simulink model "Traj_Track_twoDrones_CraneFast_ColAvo_2015b"  (R2015b)
settings: Solver=ode1  StartTime=0.0  StopTime=inf  FixedStep=T  RelTol=1e-3
StartFcn:
  | close all;
model workspace (MATLAB code in the model file):
  | T = .02; % simulation time step
values from neighbouring files (symbols this model uses):
  InitialPos_V1 = [-1 ; -1]    [CraneParam.m]
  LandFilter = ss(tf(0.3,[1 0.3]))    [CraneParam.m]
  pos_sat = 2.5    [CraneParam.m]
  radius_safe = 0.75    [CraneParam.m]
  repulsion_gain = 3.0    (= 3)    [CraneParam.m]
  repulsion_gradient = 0.2    [CraneParam.m]
  V1_gain = 0.25    [CraneParam.m]
undefined symbols (not defined in the file or in its folder): Angular, Linear, Point
libraries: robotlib x9, simulink x2, aerolibanimutils x1
settings Model: Creator=cichell2  LastModifiedBy=rmjones7
settings DataIOCC: LimitDataPoints=off  SaveFormat=Array  ReturnWorkspaceOutputs=on
settings OptimizationCC: OptimizeModelRefInitCode=on  LifeSpan=Inf  MaxStackSize=64
settings DebuggingCC: SolverPrmCheckMsg=warning
settings HardwareCC: ProdBitPerPointer=32  ProdLargestAtomicFloat=None  ProdIntDivRoundTo=Undefined  ProdEndianess=Unspecified  ProdWordSize=32  ProdHWDeviceType=Generic->Unspecified (assume 32-bit Generic)
settings RTWCC: SystemTargetFile=ert.tlc  TemplateMakefile=ert_default_tmf  Description=Embedded Coder  Toolchain=Catkin  TargetLang=C++
settings CodeAppCC: IgnoreCustomStorageClasses=off
settings ERTTargetCC: SupportContinuousTime=on
settings ConfigComp: CovModelRefEnable=Off  CovSFcnEnable=off

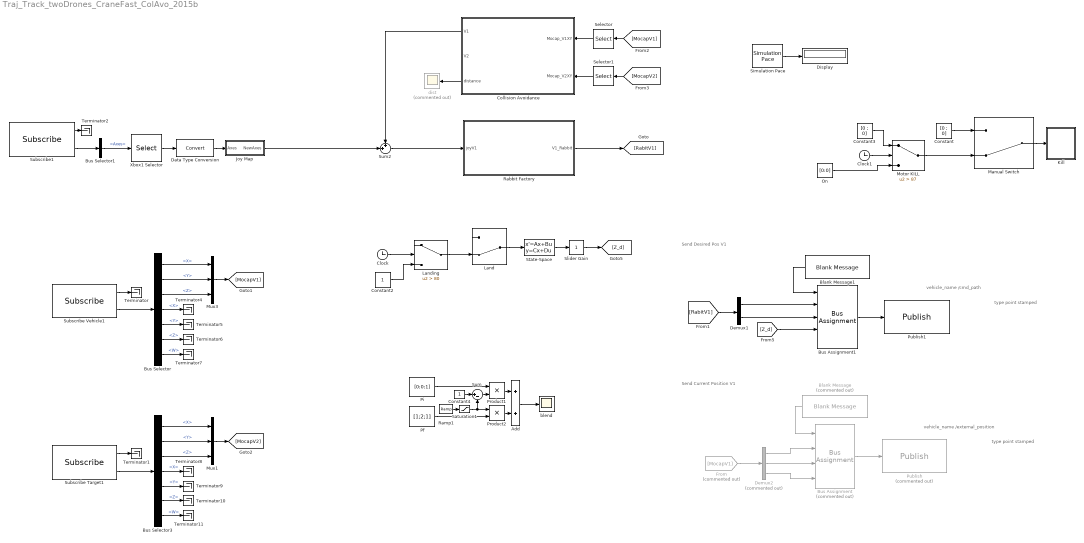
== system Traj_Track_twoDrones_CraneFast_ColAvo_2015b ==
  note: Send Desired Pos V1
  note: Send Current Position V1
  note: type point stamped
  note: vehicle_name /external_position
  note: type point stamped
  note: vehicle_name /cmd_path
  Add : Sum
  Blank Message : robotlib/Blank Message  Commented=on  SourceLibraryInfo=This block requires Robotics System Toolbox  messageType=geometry_msgs/PointStamped  SampleTime=inf
  Blank Message1 : robotlib/Blank Message  SourceLibraryInfo=This block requires Robotics System Toolbox  messageType=geometry_msgs/Twist  SampleTime=inf
  Bus Assignment : BusAssignment  Commented=on  AssignedSignals=Point.X,Point.Y,Point.Z
  Bus Assignment1 : BusAssignment  AssignedSignals=Linear.X,Linear.Y,Linear.Z,Angular.Z
  Bus Selector : BusSelector  OutputSignals=Transform.Translation.X,Transform.Translation.Y,Transform.Translation.Z,Transform.Rotation.X,Transform.Rotation.Y,Transform.Rotation.Z,Transform.Rotation.W
  Bus Selector1 : BusSelector  OutputSignals=Axes
  Bus Selector3 : BusSelector  OutputSignals=Transform.Translation.X,Transform.Translation.Y,Transform.Translation.Z,Transform.Rotation.X,Transform.Rotation.Y,Transform.Rotation.Z,Transform.Rotation.W
  Clock : Clock
  Clock1 : Clock
  Collision Avoidance : Subsystem
  Constant : Constant  Value=[0 ; 0]
  Constant2 : Constant
  Constant3 : Constant  Value=[0 ; 0]
  Constant4 : Constant
  Data Type Conversion : DataTypeConversion
  Demux1 : Demux  Outputs=2
  Demux2 : Demux  Commented=on  Outputs=3
  Display : Display
  From : From  Commented=on  GotoTag=MocapV1
  Joy Map : Subsystem
  Kill : Subsystem
  Land : ManualSwitch  CurrentSetting=0
  Landing : Switch  Criteria=u2 > Threshold  Threshold=80
  Manual Switch : ManualSwitch  CurrentSetting=0
  Motor KILL : Switch  Criteria=u2 > Threshold  Threshold=87
  Mux1 : Mux  Inputs=3
  Mux3 : Mux  Inputs=3
  On : Constant  Value=[0:0]
  Pf : Constant  Value=[1;2;1]  VectorParams1D=off
  Pi : Constant  Value=[0;0;1]  VectorParams1D=off
  Product1 : Product
  Product2 : Product
  Publish : robotlib/Publish  Commented=on  SourceLibraryInfo=This block requires Robotics System Toolbox  topicSource=Select from ROS network  topic=/crazyflie1/cmd_vel  messageType=geometry_msgs/Twist  messageQueueLength=1
  Publish1 : robotlib/Publish  SourceLibraryInfo=This block requires Robotics System Toolbox  topicSource=Select from ROS network  topic=/crazyflie1/cmd_vel  messageType=geometry_msgs/Twist  messageQueueLength=1
  Rabbit Factory : Subsystem
  Ramp1 : simulink/Sources/Ramp  slope=0.2  start=0  X0=0
  Saturation1 : Saturate  UpperLimit=1  LowerLimit=0
  Selector : Selector  InputPortWidth=3  IndexOptions=Index vector (dialog)  Indices=[1 2]  OutputSizes=1
  Selector1 : Selector  InputPortWidth=3  IndexOptions=Index vector (dialog)  Indices=[1 2]  OutputSizes=1
  Simulation Pace : aerolibanimutils/Simulation Pace  SimulationPace=1  SleepMode=MATLAB Thread  OutputPaceError=on  SampleTime=T
  Slider Gain : simulink/Math Operations/Slider Gain  low=0  gain=1  high=2
  State-Space : StateSpace  A=LandFilter.a  B=LandFilter.b  C=LandFilter.c  D=LandFilter.d  X0=-1
  Subscribe Target1 : robotlib/Subscribe  SourceLibraryInfo=This block requires Robotics System Toolbox  topicSource=Select from ROS network  topic=/vicon/Trump/Trump  messageType=geometry_msgs/TransformStamped  sampleTime=-1  messageQueueLength=1
  Subscribe Vehicle1 : robotlib/Subscribe  SourceLibraryInfo=This block requires Robotics System Toolbox  topicSource=Select from ROS network  topic=/vicon/Trump/Trump  messageType=geometry_msgs/TransformStamped  sampleTime=-1  messageQueueLength=1
  Subscribe1 : robotlib/Subscribe  SourceLibraryInfo=This block requires Robotics System Toolbox  topicSource=Select from ROS network  topic=/xbox1/joy  messageType=sensor_msgs/Joy  sampleTime=-1  messageQueueLength=1
  Sum : Sum  Inputs=|+-
  Sum2 : Sum  Inputs=++|
  Terminator{,1..2,4..11} (11 alike) : Terminator
  Xbox1 Selector : Selector  InputPortWidth=128  IndexOptions=Index vector (dialog)  Indices=[4 5]  OutputSizes=1
  blend : Scope
  dist : Scope  Commented=on
  wires:
  Simulation Pace/1 -> Display/1
  On/1 -> Motor KILL/3
  Subscribe1/2 -> Bus Selector1/1
  Xbox1 Selector/1 -> Data Type Conversion/1
  Subscribe1/1 -> Terminator2/1
  Bus Selector1/1 -> Xbox1 Selector/1  "<Axes>"
  Data Type Conversion/1 -> Joy Map/1(Axes)
  [MocapV1] -> Selector/1
  [MocapV2] -> Selector1/1
  State-Space/1 -> Slider Gain/1
  Clock/1 -> Landing/2
  Constant2/1 -> Landing/3
  Clock1/1 -> Motor KILL/2
  Constant3/1 -> Motor KILL/1
  Constant/1 -> Manual Switch/1
  Motor KILL/1 -> Manual Switch/2
  Landing/1 -> Land/2
  Land/1 -> State-Space/1
  Bus Assignment/1 -> Publish/1
  Subscribe Vehicle1/2 -> Bus Selector/1
  Subscribe Vehicle1/1 -> Terminator/1
  Bus Selector/4 -> Terminator4/1  "<X>"
  Bus Selector/1 -> Mux3/1  "<X>"
  Bus Selector/3 -> Mux3/3  "<Z>"
  Bus Selector/6 -> Terminator6/1  "<Z>"
  Bus Selector/7 -> Terminator7/1  "<W>"
  Bus Selector/5 -> Terminator5/1  "<Y>"
  Bus Selector/2 -> Mux3/2  "<Y>"
  Subscribe Target1/2 -> Bus Selector3/1
  Subscribe Target1/1 -> Terminator1/1
  Bus Selector3/4 -> Terminator8/1  "<X>"
  Bus Selector3/6 -> Terminator10/1  "<Z>"
  Bus Selector3/7 -> Terminator11/1  "<W>"
  Bus Selector3/5 -> Terminator9/1  "<Y>"
  Sum2/1 -> Rabbit Factory/1(joyV1)
  Joy Map/1(NewAxes) -> Sum2/2
  Collision Avoidance/1(V1) -> Sum2/1
  Collision Avoidance/3(distance) -> dist/1
  Slider Gain/1 -> [Z_d]
  Manual Switch/1 -> Kill/Trigger
  Rabbit Factory/1(V1_Rabbit) -> [RabitV1]
  Bus Assignment1/1 -> Publish1/1
  Blank Message1/1 -> Bus Assignment1/1
  [Z_d] -> Bus Assignment1/4
  [RabitV1] -> Demux1/1
  Demux1/1 -> Bus Assignment1/2
  Demux1/2 -> Bus Assignment1/3
  Blank Message/1 -> Bus Assignment/1
  Mux3/1 -> [MocapV1]
  Selector/1 -> Collision Avoidance/1(Mocap_V1XY)
  Selector1/1 -> Collision Avoidance/2(Mocap_V2XY)
  Bus Selector3/1 -> Mux1/1  "<X>"
  Bus Selector3/3 -> Mux1/3  "<Z>"
  Bus Selector3/2 -> Mux1/2  "<Y>"
  Mux1/1 -> [MocapV2]
  Demux2/2 -> Bus Assignment/3
  Demux2/1 -> Bus Assignment/2
  Demux2/3 -> Bus Assignment/4
  From/1 -> Demux2/1
  Ramp1/1 -> Saturation1/1
  Product1/1 -> Add/1
  Product2/1 -> Add/2
  Pi/1 -> Product1/1
  Pf/1 -> Product2/2
  Constant4/1 -> Sum/1
  Sum/1 -> Product1/2
  Saturation1/1 -> Product2/1, Sum/2
  Add/1 -> blend/1

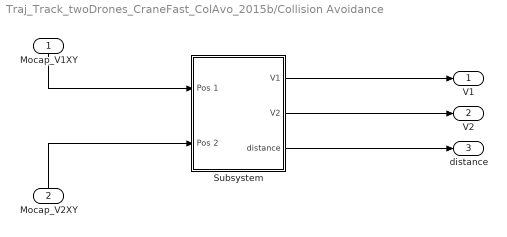
== system Traj_Track_twoDrones_CraneFast_ColAvo_2015b/Collision Avoidance ==
  Mocap_V1XY : Inport
  Mocap_V2XY : Inport  Port=2
  Subsystem : Subsystem
  V1 : Outport
  V2 : Outport  Port=2
  distance : Outport  Port=3
  wires:
  Subsystem/1(V1) -> V1/1
  Mocap_V2XY/1 -> Subsystem/2(Pos 2)
  Mocap_V1XY/1 -> Subsystem/1(Pos 1)
  Subsystem/2(V2) -> V2/1
  Subsystem/3(distance) -> distance/1

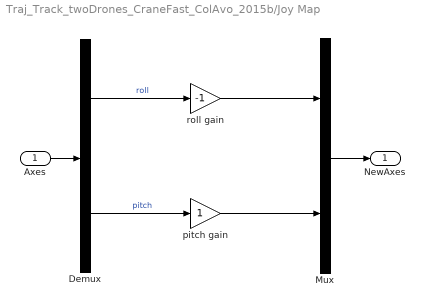
== system Traj_Track_twoDrones_CraneFast_ColAvo_2015b/Joy Map ==
  Axes : Inport
  Demux : Demux  Outputs=2
  Mux : Mux  Inputs=2
  pitch gain : Gain
  roll gain : Gain  Gain=-1
  NewAxes : Outport
  wires:
  Axes/1 -> Demux/1
  Mux/1 -> NewAxes/1
  Demux/2 -> pitch gain/1  "pitch"
  Demux/1 -> roll gain/1  "roll"
  roll gain/1 -> Mux/1
  pitch gain/1 -> Mux/2

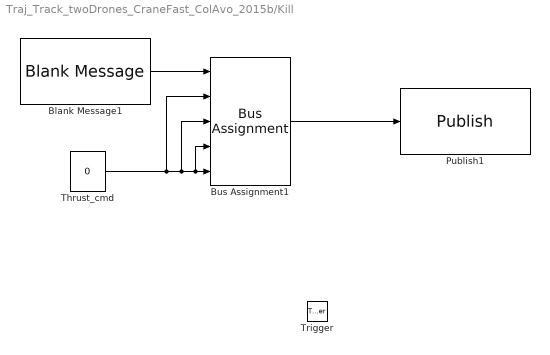
== system Traj_Track_twoDrones_CraneFast_ColAvo_2015b/Kill ==
  Trigger : TriggerPort  PortDimensions=1
  Blank Message1 : robotlib/Blank Message  SourceLibraryInfo=This block requires Robotics System Toolbox  messageType=geometry_msgs/Twist  SampleTime=inf
  Bus Assignment1 : BusAssignment  AssignedSignals=Linear.X,Linear.Y,Linear.Z,Angular.Z
  Publish1 : robotlib/Publish  SourceLibraryInfo=This block requires Robotics System Toolbox  topicSource=Select from ROS network  topic=/crazyflie1/cmd_vel  messageType=geometry_msgs/Twist  messageQueueLength=1
  Thrust_cmd : Constant  Value=0
  wires:
  Thrust_cmd/1 -> Bus Assignment1/2, Bus Assignment1/3, Bus Assignment1/4, Bus Assignment1/5
  Blank Message1/1 -> Bus Assignment1/1
  Bus Assignment1/1 -> Publish1/1

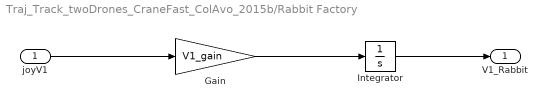
== system Traj_Track_twoDrones_CraneFast_ColAvo_2015b/Rabbit Factory ==
  joyV1 : Inport
  Gain : Gain  Gain=V1_gain
  Integrator : Integrator  InitialCondition=InitialPos_V1  LimitOutput=on  UpperSaturationLimit=pos_sat  LowerSaturationLimit=-pos_sat
  V1_Rabbit : Outport
  wires:
  Integrator/1 -> V1_Rabbit/1
  Gain/1 -> Integrator/1
  joyV1/1 -> Gain/1

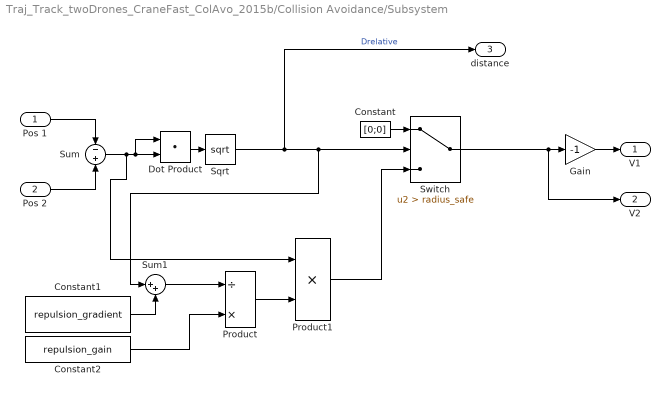
== system Traj_Track_twoDrones_CraneFast_ColAvo_2015b/Collision Avoidance/Subsystem ==
  Pos 1 : Inport
  Pos 2 : Inport  Port=2
  Constant : Constant  Value=[0;0]
  Constant1 : Constant  Value=repulsion_gradient
  Constant2 : Constant  Value=repulsion_gain
  Dot Product : DotProduct  InputSameDT=on  OutDataTypeStr=Inherit: Inherit via internal rule
  Gain : Gain  Gain=-1
  Product : Product  Inputs=/*
  Product1 : Product
  Sqrt : Sqrt  SaturateOnIntegerOverflow=on
  Sum : Sum  Inputs=-+
  Sum1 : Sum  Inputs=|++
  Switch : Switch  Criteria=u2 > Threshold  Threshold=radius_safe
  V1 : Outport
  V2 : Outport  Port=2
  distance : Outport  Port=3
  wires:
  Pos 1/1 -> Sum/1
  Pos 2/1 -> Sum/2
  Dot Product/1 -> Sqrt/1
  Gain/1 -> V1/1
  Sqrt/1 -> Sum1/1, Switch/2, distance/1  "Drelative"
  Constant/1 -> Switch/1
  Switch/1 -> V2/1, Gain/1
  Sum/1 -> Product1/1, Dot Product/1, Dot Product/2
  Sum1/1 -> Product/1
  Constant1/1 -> Sum1/2
  Product/1 -> Product1/2
  Product1/1 -> Switch/3
  Constant2/1 -> Product/2
